simulink model "Udan_SOC"  (R2017b)
settings: Solver=FixedStepAuto  StartTime=0.0  StopTime=1000  FixedStep=0.1  RelTol=1e-3
values from neighbouring files (symbols this model uses):
  DenominatorOfIntegratorFactor = 100.0    [SOC_Stateflow.sldd]
  SOC_CalcSohLKT = 1.0    [SOC_Stateflow.sldd]
  SOC_CalcSOHTempLimit = 70.0    [SOC_Stateflow.sldd]
  SOC_CapPerCycle = 100.0    [SOC_Stateflow.sldd]
  SOC_CapTemp_HLimit = 200.0    [SOC_Stateflow.sldd]
  SOC_CapTemp_LLimit = 0.0    [SOC_Stateflow.sldd]
  Soc_ConfigInfo = 0    [SOC_Stateflow.sldd]
  SOC_DchgEndCalib = 0.0    [SOC_Stateflow.sldd]
  SOC_DiffVoltMin = 10.0    [SOC_Stateflow.sldd]
  SOC_DSOCJumpMax = 500.0    [SOC_Stateflow.sldd]
  SOC_EfficientHighLimit = 250.0    [SOC_Stateflow.sldd]
  SOC_EfficientLowLimit = 40.0    [SOC_Stateflow.sldd]
  SOC_EmptyAus = 0.0    [SOC_Stateflow.sldd]
  SOC_EnableOcv = 1.0    [SOC_Stateflow.sldd]
  SOC_END_CALIB_STATE : value not decoded    [SOC_Stateflow.sldd]
  SOC_HighRealSoc = 95.0    [SOC_Stateflow.sldd]
  SOC_LKTSohCycles = 0.0 1.0 10.0 20.0 30.0 40.0 50.0 60.0 70.0 80.0 90.0 100.0 110.0 120.0 130.0 140.0 150.0 160.0 170.0 180.0 190.0 200.0 210.0 220.0 230.0 240.0 250.0 260.0 270.0 280.0 290.0 300.0 310.0 320.0 330.0 340.0 350.0 360.0 370.0 380.0 390.0 400.0 410.0 420.0 430.0 440.0 450.0 460.0 470.0 480.0 490.0 500.0 510.0 520.0 530.0 540.0 550.0 560.0 570.0 580.0 590.0 600.0 610.0 620.0 630.0 640.0 650.0 660.0 670.0    [SOC_Stateflow.sldd]
  SOC_LKTSohTable = 1000.0 991.0 989.0 992.0 993.0 995.0 994.0 993.0 1000.0 997.0 1002.0 1000.0 992.0 1000.0 989.0 992.0 989.0 994.0 989.0 993.0 994.0 994.0 994.0 993.0 991.0 991.0 992.0 993.0 991.0 985.0 985.0 985.0 979.0 975.0 978.0 984.0 982.0 974.0 975.0 972.0 972.0 975.0 977.0 977.0 974.0 971.0 973.0 971.0 966.0 968.0 965.0 959.0 957.0 956.0 957.0 954.0 955.0 951.0 954.0 951.0 942.0 942.0 940.0 942.0 947.0 949.0    [SOC_Stateflow.sldd]
  SOC_LowRealSoc = 5.0    [SOC_Stateflow.sldd]
  SOC_NominalCap_AmS = 576000000.0    [SOC_Stateflow.sldd]
  SOC_NominalVol = 4000.0    [SOC_Stateflow.sldd]
  SOC_OCVTemp_HLimit = 106.0    [SOC_Stateflow.sldd]
  SOC_OCVTemp_LLimit = 29.0    [SOC_Stateflow.sldd]
  SOC_ShortCalibDSoc = 1.0    [SOC_Stateflow.sldd]
  SOC_SOCResolution = 10000.0    [SOC_Stateflow.sldd]
  SOC_SohCalcCapPercent = 8.0    [SOC_Stateflow.sldd]
  SOC_SohCalcHighLimit = 60.0    [SOC_Stateflow.sldd]
  SOC_SohCalcLowLimit = 10.0    [SOC_Stateflow.sldd]
  SOC_SohCalcMidLimit = 30.0    [SOC_Stateflow.sldd]
  SOC_SOHResolution = 1000.0    [SOC_Stateflow.sldd]
  SOC_State = <binary blob, 1163 chars, not shown>    [SOC_Stateflow.sldd]
  SOC_TempCap_CapBuffer : value not decoded    [SOC_Stateflow.sldd]
  SOC_TempCap_TempBuffer : value not decoded    [SOC_Stateflow.sldd]
  SocOcvCalib_ConfigInfo = 0.0    [SOC_Stateflow.sldd]
  SocOcvCalib_SocBuffer1 : value not decoded    [SOC_Stateflow.sldd]
  SocOcvCalib_TempBuffer : value not decoded    [SOC_Stateflow.sldd]
  SocOcvCalib_VoltageBuffer1 = 3300.0 3303.0 3305.0 3307.0 3310.0 3311.0 3313.0 3314.0 3316.0 3317.0 3319.0 3320.0 3322.0 3323.0 3325.0 3322.0 3323.0 3325.0 3310.0 3313.0 3315.0 3317.0 3320.0 3321.0 3323.0 3324.0 3326.0 3327.0 3329.0 3330.0 3332.0 3333.0 3335.0 3332.0 3333.0 3335.0 3320.0 3323.0 3325.0 3327.0 3330.0 3331.0 3333.0 3334.0 3336.0 3337.0 3339.0 3340.0 3342.0 3343.0 3345.0 3342.0 3343.0 3345.0 3330.0 3333.0 3335.0 3    [SOC_Stateflow.sldd]
  SOHCalibCycle = 10.0    [SOC_Stateflow.sldd]
undefined symbols (not defined in the file or in its folder): DatetimeM_GetReturnType, ParameterM_EeepParaIndexType, Soc_CumuLativeTypeType, SOC_EgthTempChgValue, Soc_EnergyBuffer, SOC_FithTempChgValue, SOC_FstSlowTempChgValue, SOC_FstTempChgValue, SOC_FthTempChgValue, SOC_MaxCap_AmS, SOC_SethTempChgValue, SOC_SixTempChgValue, SOC_SndSlowTempChgValue, SOC_SndTempChgValue, SOC_TrdSlowTempChgValue, SOC_TrdTempChgValue, SocDiagCalib_NoCalibReasonType
libraries: simulink x138, hdlsllib x24, dspindex x4
(part 8 of 10)

== system Udan_SOC/SOC_Calculate/UdanSOCCalcn/WriteSOH/Enabled Subsystem4 ==
  index : Inport
  data : Inport  Port=2
  Enable : EnablePort
  Abs : Abs
  Add : Sum  Inputs=+-  AccumDataTypeStr=int32  OutDataTypeStr=int32
  Constant : Constant  Value=20  OutDataTypeStr=uint8
  Divide : Product  Inputs=*/  OutDataTypeStr=uint32
  Logical Operator : Logic  Operator=OR  AllPortsSameDT=off  OutDataTypeStr=boolean
  Relational Operator : RelationalOperator  OutDataTypeStr=boolean  RndMeth=Simplest
  S-Function1 : S-Function  FunctionName=sfn_NVMRead  SFunctionDeploymentMode=off  EnableBusSupport=off
  EeepWriteFailure : Outport
  wires:
  index/1 -> S-Function1/1
  Logical Operator/1 -> EeepWriteFailure/1
  Abs/1 -> Relational Operator/1
  Relational Operator/1 -> Logical Operator/2
  Constant/1 -> Divide/2
  S-Function1/2 -> Add/1
  Add/1 -> Abs/1
  Divide/1 -> Relational Operator/2
  data/1 -> Divide/1, Add/2
  S-Function1/1 -> Logical Operator/1

== system Udan_SOC/SOC_Calculate/UdanSOCCalcn/WriteSOH/Enabled Subsystem5 ==
  index : Inport
  data : Inport  Port=2
  Enable : EnablePort
  Abs : Abs
  Add : Sum  Inputs=+-  AccumDataTypeStr=int32  OutDataTypeStr=int32
  Constant : Constant  Value=20  OutDataTypeStr=uint8
  Divide : Product  Inputs=*/  OutDataTypeStr=uint32
  Logical Operator : Logic  Operator=OR  AllPortsSameDT=off  OutDataTypeStr=boolean
  Relational Operator : RelationalOperator  OutDataTypeStr=boolean  RndMeth=Simplest
  S-Function1 : S-Function  FunctionName=sfn_NVMRead  SFunctionDeploymentMode=off  EnableBusSupport=off
  EeepWriteFailure : Outport
  wires:
  index/1 -> S-Function1/1
  Logical Operator/1 -> EeepWriteFailure/1
  Abs/1 -> Relational Operator/1
  Relational Operator/1 -> Logical Operator/2
  Constant/1 -> Divide/2
  S-Function1/2 -> Add/1
  Add/1 -> Abs/1
  Divide/1 -> Relational Operator/2
  data/1 -> Divide/1, Add/2
  S-Function1/1 -> Logical Operator/1

== system Udan_SOC/SOC_Calculate/UdanSOCCalcn/WriteSOH/Enabled Subsystem6 ==
  index : Inport
  data : Inport  Port=2
  Enable : EnablePort
  Abs : Abs
  Add : Sum  Inputs=+-  AccumDataTypeStr=int32  OutDataTypeStr=int32
  Constant : Constant  Value=20  OutDataTypeStr=uint8
  Divide : Product  Inputs=*/  OutDataTypeStr=uint32
  Logical Operator : Logic  Operator=OR  AllPortsSameDT=off  OutDataTypeStr=boolean
  Relational Operator : RelationalOperator  OutDataTypeStr=boolean  RndMeth=Simplest
  S-Function1 : S-Function  FunctionName=sfn_NVMRead  SFunctionDeploymentMode=off  EnableBusSupport=off
  EeepWriteFailure : Outport
  wires:
  index/1 -> S-Function1/1
  Logical Operator/1 -> EeepWriteFailure/1
  Abs/1 -> Relational Operator/1
  Relational Operator/1 -> Logical Operator/2
  Constant/1 -> Divide/2
  S-Function1/2 -> Add/1
  Add/1 -> Abs/1
  Divide/1 -> Relational Operator/2
  data/1 -> Divide/1, Add/2
  S-Function1/1 -> Logical Operator/1

== system Udan_SOC/SOC_Calculate/UdanSOCCalcn/WriteSOH/Enabled Subsystem7 ==
  index : Inport
  data : Inport  Port=2
  Enable : EnablePort
  Abs : Abs
  Add : Sum  Inputs=+-  AccumDataTypeStr=int32  OutDataTypeStr=int32
  Constant : Constant  Value=20  OutDataTypeStr=uint8
  Divide : Product  Inputs=*/  OutDataTypeStr=uint32
  Logical Operator : Logic  Operator=OR  AllPortsSameDT=off  OutDataTypeStr=boolean
  Relational Operator : RelationalOperator  OutDataTypeStr=boolean  RndMeth=Simplest
  S-Function1 : S-Function  FunctionName=sfn_NVMRead  SFunctionDeploymentMode=off  EnableBusSupport=off
  EeepWriteFailure : Outport
  wires:
  index/1 -> S-Function1/1
  Logical Operator/1 -> EeepWriteFailure/1
  Abs/1 -> Relational Operator/1
  Relational Operator/1 -> Logical Operator/2
  Constant/1 -> Divide/2
  S-Function1/2 -> Add/1
  Add/1 -> Abs/1
  Divide/1 -> Relational Operator/2
  data/1 -> Divide/1, Add/2
  S-Function1/1 -> Logical Operator/1

== system Udan_SOC/SOC_Calculate/UdanSOCCalcn/CalcChgSOH/Subsystem1/Subsystem ==
  HighIndex : Inport
  LowIndex : Inport  Port=2
  Enable : EnablePort
  Add : Sum
  Bit Rotate : hdlsllib/Logic and Bit Operations/Bit Rotate  mode=Rotate Left  N=16
      settings: SourceProductName=HDL Coder  SourceProductBaseCode=HD
  Data Type Conversion : DataTypeConversion  OutDataTypeStr=uint32
  soc : Outport
  wires:
  LowIndex/1 -> Add/2
  Bit Rotate/1 -> Add/1
  Data Type Conversion/1 -> Bit Rotate/1
  HighIndex/1 -> Data Type Conversion/1
  Add/1 -> soc/1  "soc"

== system Udan_SOC/SOC_Calculate/UdanSOCCalcn/CalcDchgSOH/Subsystem1/Subsystem ==
  HighIndex : Inport
  LowIndex : Inport  Port=2
  Enable : EnablePort
  Add : Sum
  Bit Rotate : hdlsllib/Logic and Bit Operations/Bit Rotate  mode=Rotate Left  N=16
      settings: SourceProductName=HDL Coder  SourceProductBaseCode=HD
  Data Type Conversion : DataTypeConversion  OutDataTypeStr=uint32
  soc : Outport
  wires:
  LowIndex/1 -> Add/2
  Bit Rotate/1 -> Add/1
  Data Type Conversion/1 -> Bit Rotate/1
  HighIndex/1 -> Data Type Conversion/1
  Add/1 -> soc/1  "soc"

== system Udan_SOC/SOC_Calculate/UdanSOCCalcn/CapAdder1/Enabled Subsystem1/Enabled Subsystem1 ==
  CellLowTemp : Inport
  UCell : Inport  Port=2
  CalcSoc : Inport  Port=3
  soh : Inport  Port=4
  Enable : EnablePort
  CalcLeftCap : Subsystem
  Constant11 : Constant  Value=SocOcvCalib_VoltageBuffer1
  Constant12 : Constant  Value=SocOcvCalib_SocBuffer1
  Constant2 : Constant  Value=20  OutDataTypeStr=uint16
  Constant3 : Constant  Value=SocOcvCalib_TempBuffer  OutDataTypeStr=uint8
  Constant6 : Constant  Value=92160  OutDataTypeStr=uint32
  Logical Operator : Logic  Operator=NOT  AllPortsSameDT=off  OutDataTypeStr=boolean
  Lookup Table Dynamic1 : simulink/Lookup Tables/Lookup Table Dynamic  LookUpMeth=Interpolation-Use End Values  OutDataType=fixdt('uint16')  OutScaling=[]  OutputDataTypeScalingMode=Specify via dialog  OutDataTypeStr=uint16  DoSatur=on
      settings: SourceProductName=Simulink
  Lookup Table Dynamic2 : simulink/Lookup Tables/Lookup Table Dynamic  LookUpMeth=Use Input Nearest  OutDataType=fixdt('uint8')  OutScaling=[]  OutputDataTypeScalingMode=Specify via dialog  OutDataTypeStr=uint8  DoSatur=on
      settings: SourceProductName=Simulink
  MATLAB Function : MATLAB Function  TreatAsAtomicUnit=on
  Relational Operator2 : RelationalOperator  OutDataTypeStr=boolean  RndMeth=Simplest
  Switch : Switch  Criteria=u2 > Threshold
  Variable Selector : dspindex/Variable Selector  NumInputs=1  rowsOrCols=Rows  IdxMode=Variable  Elements=[1 3]  ZerOneIdxMode=One-based  errmode=Clip Index  FillMode=on  FillValues=0
  LKTSOC : Outport
  LeftCap2 : Outport  Port=2
  wires:
  CellLowTemp/1 -> Lookup Table Dynamic2/1, CalcLeftCap/2(CellLowTemp)
  UCell/1 -> Lookup Table Dynamic1/1
  Lookup Table Dynamic2/1 -> Variable Selector/2
  MATLAB Function/1(y) -> Lookup Table Dynamic2/3
  Constant3/1 -> MATLAB Function/1(u), Lookup Table Dynamic2/2
  Constant12/1 -> Lookup Table Dynamic1/3
  Variable Selector/1 -> Lookup Table Dynamic1/2
  Lookup Table Dynamic1/1 -> LKTSOC/1, CalcLeftCap/1(soc), Relational Operator2/1  "soc"
  Relational Operator2/1 -> Logical Operator/1, CalcLeftCap/Enable
  Switch/1 -> LeftCap2/1
  Constant2/1 -> Relational Operator2/2
  Constant6/1 -> Switch/1  "soc"
  Logical Operator/1 -> Switch/2
  CalcLeftCap/1(Soc) -> Switch/3
  CalcSoc/1 -> CalcLeftCap/3(CalcSoc)
  soh/1 -> CalcLeftCap/4(soh)
  Constant11/1 -> Variable Selector/1

== system Udan_SOC/SOC_Calculate/UdanSOCCalcn/CapAdder1/Enabled Subsystem1/Function-Call Subsystem ==
  function : TriggerPort  TriggerType=function-call  VariantControl=Variant
  sfn_SetLowPower : S-Function  FunctionName=sfn_SetLowPower  SFunctionDeploymentMode=off  EnableBusSupport=off  mask(Legacy Function){SFunctionSpec=void UserSetLowPowerFlg(void), ShowSpec=on}
      mask prompts: ShowSpec "Display function specification"
      mask help:
      | This block allows you to call the legacy functions specified by the following Legacy Code Tool definition:
      | def.SFunctionName = 'sfn_SetLowPower';
      | def.OutputFcnSpec = 'void UserSetLowPowerFlg(void)';
      | def.HeaderFiles = {'PowerM.h'};
      mask Help: <p>This block was generated automatically by the Legacy Code Tool. For detailed help on this tool, call<a href="matlab:legacy_code('help')"> legacy_code('help')</a>.</p>
      mask Callback ShowSpec:
      | if strcmp(get_param(gcbh, 'ShowSpec'), 'on')
      |   set_param(gcbh, 'MaskDisplay', sprintf('fprintf(''%s'');', get_param(gcbh, 'SFunctionSpec')));
      | else
      |   set_param(gcbh, 'MaskDisplay', sprintf('fprintf(''%s'');', get_param(gcbh, 'FunctionName')));
      | end
      mask Display: fprintf('void UserSetLowPowerFlg(void)');

== system Udan_SOC/SOC_Calculate/UdanSOCCalcn/CapAdder1/LKT/LKT_Temp20 ==
  Cur : Inport
  UCell : Inport  Port=2
  Enable : EnablePort
  Constant : Constant  Value=1000  OutDataTypeStr=uint16
  Constant1 : Constant  Value=1000  OutDataTypeStr=uint16
  Constant2 : Constant  Value=500  OutDataTypeStr=uint16
  Constant3 : Constant  Value=0  OutDataTypeStr=uint8
  Current_1C : Subsystem  TreatAsAtomicUnit=on
  Current_1C1 : Subsystem  TreatAsAtomicUnit=on
  Logical Operator : Logic  AllPortsSameDT=off  OutDataTypeStr=boolean
  Logical Operator1 : Logic  Operator=NOT  AllPortsSameDT=off  OutDataTypeStr=boolean
  Logical Operator2 : Logic  Operator=NOT  AllPortsSameDT=off  OutDataTypeStr=boolean
  Relational Operator : RelationalOperator  OutDataTypeStr=boolean  RndMeth=Simplest
  Relational Operator1 : RelationalOperator  Operator=<  OutDataTypeStr=boolean  RndMeth=Simplest
  Relational Operator2 : RelationalOperator  OutDataTypeStr=boolean  RndMeth=Simplest
  Switch : Switch  Criteria=u2 > Threshold
  Switch1 : Switch  Criteria=u2 > Threshold
  SOC : Outport
  wires:
  Constant/1 -> Relational Operator/2
  Relational Operator/1 -> Logical Operator2/1, Current_1C/Enable
  UCell/1 -> Current_1C1/1(UCell), Current_1C/1(UCell)
  Constant1/1 -> Relational Operator1/2
  Constant2/1 -> Relational Operator2/2
  Relational Operator1/1 -> Logical Operator/1
  Relational Operator2/1 -> Logical Operator/2
  Logical Operator/1 -> Logical Operator1/1, Current_1C1/Enable
  Cur/1 -> Relational Operator/1, Relational Operator1/1, Relational Operator2/1
  Logical Operator1/1 -> Switch/2
  Current_1C1/1(SOC) -> Switch/3
  Logical Operator2/1 -> Switch1/2
  Current_1C/1(SOC) -> Switch1/3
  Switch1/1 -> Switch/1
  Constant3/1 -> Switch1/1
  Switch/1 -> SOC/1

== system Udan_SOC/SOC_Calculate/UdanSOCCalcn/CapAdder1/LKT/LKT_Temp40 ==
  Cur : Inport
  UCell : Inport  Port=2
  Enable : EnablePort
  Constant1 : Constant  Value=500  OutDataTypeStr=uint16
  Constant2 : Constant  Value=200  OutDataTypeStr=uint16
  Constant3 : Constant  Value=500  OutDataTypeStr=uint16
  Constant4 : Constant  Value=0  OutDataTypeStr=uint8
  Constant6 : Constant  Value=4118  OutDataTypeStr=uint16
  Current_1C : Subsystem  TreatAsAtomicUnit=on
  Current_1C1 : Subsystem  TreatAsAtomicUnit=on
  Logical Operator : Logic  Inputs=3  AllPortsSameDT=off  OutDataTypeStr=boolean
  Logical Operator1 : Logic  Operator=NOT  AllPortsSameDT=off  OutDataTypeStr=boolean
  Logical Operator2 : Logic  Operator=NOT  AllPortsSameDT=off  OutDataTypeStr=boolean
  Relational Operator1 : RelationalOperator  Operator=<  OutDataTypeStr=boolean  RndMeth=Simplest
  Relational Operator2 : RelationalOperator  OutDataTypeStr=boolean  RndMeth=Simplest
  Relational Operator3 : RelationalOperator  OutDataTypeStr=boolean  RndMeth=Simplest
  Relational Operator4 : RelationalOperator  OutDataTypeStr=boolean  RndMeth=Simplest
  Switch : Switch  Criteria=u2 > Threshold
  Switch1 : Switch  Criteria=u2 > Threshold
  SOC : Outport
  wires:
  Cur/1 -> Relational Operator1/1, Relational Operator2/1, Relational Operator3/1
  Constant1/1 -> Relational Operator1/2
  Relational Operator2/1 -> Logical Operator/2
  Relational Operator1/1 -> Logical Operator/1
  Constant2/1 -> Relational Operator2/2
  Constant3/1 -> Relational Operator3/2
  Relational Operator3/1 -> Logical Operator2/1, Current_1C/Enable
  UCell/1 -> Current_1C1/1(UCell), Relational Operator4/1, Current_1C/1(UCell)
  Logical Operator1/1 -> Switch/2
  Switch1/1 -> Switch/1
  Switch/1 -> SOC/1
  Constant4/1 -> Switch1/1
  Current_1C/1(SOC) -> Switch1/3
  Current_1C1/1(SOC) -> Switch/3
  Logical Operator2/1 -> Switch1/2
  Logical Operator/1 -> Logical Operator1/1, Current_1C1/Enable
  Constant6/1 -> Relational Operator4/2
  Relational Operator4/1 -> Logical Operator/3

== system Udan_SOC/SOC_Calculate/UdanSOCCalcn/CapAdder1/LKT/LKT_Temp45 ==
  Cur : Inport
  UCell : Inport  Port=2
  Enable : EnablePort
  Constant1 : Constant  Value=175  OutDataTypeStr=uint16
  Constant2 : Constant  Value=100  OutDataTypeStr=uint16
  Constant3 : Constant  Value=250  OutDataTypeStr=uint16
  Constant4 : Constant  Value=0  OutDataTypeStr=uint8
  Current_1C : Subsystem  TreatAsAtomicUnit=on
  Current_1C1 : Subsystem  TreatAsAtomicUnit=on
  Logical Operator : Logic  AllPortsSameDT=off  OutDataTypeStr=boolean
  Logical Operator1 : Logic  Operator=NOT  AllPortsSameDT=off  OutDataTypeStr=boolean
  Logical Operator2 : Logic  Operator=NOT  AllPortsSameDT=off  OutDataTypeStr=boolean
  Relational Operator1 : RelationalOperator  Operator=<  OutDataTypeStr=boolean  RndMeth=Simplest
  Relational Operator2 : RelationalOperator  OutDataTypeStr=boolean  RndMeth=Simplest
  Relational Operator3 : RelationalOperator  Operator=>  OutDataTypeStr=boolean  RndMeth=Simplest
  Switch : Switch  Criteria=u2 > Threshold
  Switch1 : Switch  Criteria=u2 > Threshold
  SOC : Outport
  wires:
  Relational Operator3/1 -> Logical Operator2/1, Current_1C/Enable
  UCell/1 -> Current_1C1/1(UCell), Current_1C/1(UCell)
  Cur/1 -> Relational Operator2/1, Relational Operator1/1, Relational Operator3/1
  Constant3/1 -> Relational Operator3/2
  Current_1C/1(SOC) -> Switch1/3
  Current_1C1/1(SOC) -> Switch/3
  Constant1/1 -> Relational Operator1/2
  Relational Operator2/1 -> Logical Operator/2
  Switch/1 -> SOC/1
  Logical Operator/1 -> Logical Operator1/1, Current_1C1/Enable
  Constant4/1 -> Switch1/1
  Logical Operator1/1 -> Switch/2
  Switch1/1 -> Switch/1
  Relational Operator1/1 -> Logical Operator/1
  Logical Operator2/1 -> Switch1/2
  Constant2/1 -> Relational Operator2/2

== system Udan_SOC/SOC_Calculate/UdanSOCCalcn/Function-Call Subsystem4/Subsystem1/Subsystem ==
  HighIndex : Inport
  LowIndex : Inport  Port=2
  Enable : EnablePort
  Add : Sum
  Bit Rotate : hdlsllib/Logic and Bit Operations/Bit Rotate  mode=Rotate Left  N=16
      settings: SourceProductName=HDL Coder  SourceProductBaseCode=HD
  Data Type Conversion : DataTypeConversion  OutDataTypeStr=uint32
  soc : Outport
  wires:
  LowIndex/1 -> Add/2
  Bit Rotate/1 -> Add/1
  Data Type Conversion/1 -> Bit Rotate/1
  HighIndex/1 -> Data Type Conversion/1
  Add/1 -> soc/1  "soc"

== system Udan_SOC/SOC_Calculate/UdanSOCCalcn/Function-Call Subsystem4/Subsystem1/Subsystem1 ==
  HighIndex : Inport
  LowIndex : Inport  Port=2
  DefaultValue : Inport  Port=3
  Enable : EnablePort
  Constant1 : Constant  Value=0  OutDataTypeStr=uint8
  Constant2 : Constant  Value=0  OutDataTypeStr=uint8
  Logical Operator : Logic  AllPortsSameDT=off  OutDataTypeStr=boolean
  Logical Operator1 : Logic  Operator=NOT  AllPortsSameDT=off  OutDataTypeStr=boolean
  Relational Operator : RelationalOperator  Operator===  OutDataTypeStr=boolean  RndMeth=Simplest
  Relational Operator1 : RelationalOperator  Operator===  OutDataTypeStr=boolean  RndMeth=Simplest
  S-Function : S-Function  FunctionName=sfn_NVMRead  SFunctionDeploymentMode=off  EnableBusSupport=off
  S-Function1 : S-Function  FunctionName=sfn_NVMRead  SFunctionDeploymentMode=off  EnableBusSupport=off
  Subsystem : Subsystem
  Switch : Switch  Criteria=u2 > Threshold
  EeepRead32 : Outport
  wires:
  DefaultValue/1 -> Switch/1
  [ReadLowOk] -> Logical Operator/1
  S-Function/2 -> Subsystem/1(HighIndex)
  S-Function/1 -> Relational Operator/1
  S-Function1/2 -> Subsystem/2(LowIndex)
  HighIndex/1 -> S-Function/1
  Constant1/1 -> Relational Operator/2
  Constant2/1 -> Relational Operator1/2
  LowIndex/1 -> S-Function1/1
  Relational Operator/1 -> Logical Operator/2
  Logical Operator/1 -> Logical Operator1/1, Subsystem/Enable
  Relational Operator1/1 -> [ReadLowOk]
  S-Function1/1 -> Relational Operator1/1
  Subsystem/1(soc) -> Switch/3
  Logical Operator1/1 -> Switch/2
  Switch/1 -> EeepRead32/1

== system Udan_SOC/SOC_Calculate/UdanSOCCalcn/Function-Call Subsystem4/Subsystem2/Subsystem ==
  data : Inport
  HighIndex : Inport  Port=2
  LowIndex : Inport  Port=3
  Bit Rotate : hdlsllib/Logic and Bit Operations/Bit Rotate  mode=Rotate Right  N=16
      settings: SourceProductName=HDL Coder  SourceProductBaseCode=HD
  Data Type Conversion : DataTypeConversion  OutDataTypeStr=uint16
  Data Type Conversion1 : DataTypeConversion  OutDataTypeStr=uint16
  S-Function : S-Function  FunctionName=sfn_NVMWrite  SFunctionDeploymentMode=off  EnableBusSupport=off
  S-Function1 : S-Function  FunctionName=sfn_NVMWrite  SFunctionDeploymentMode=off  EnableBusSupport=off
  Terminator : Terminator
  Terminator1 : Terminator
  wires:
  data/1 -> Data Type Conversion1/1, Bit Rotate/1
  Data Type Conversion/1 -> S-Function/2
  S-Function1/1 -> Terminator1/1
  Bit Rotate/1 -> Data Type Conversion/1
  Data Type Conversion1/1 -> S-Function1/2
  S-Function/1 -> Terminator/1
  HighIndex/1 -> S-Function/1
  LowIndex/1 -> S-Function1/1

== system Udan_SOC/SOC_Calculate/UdanSOCCalcn/LKTSOC/Subsystem1/Subsystem ==
  HighIndex : Inport
  LowIndex : Inport  Port=2
  Enable : EnablePort
  Add : Sum
  Bit Rotate : hdlsllib/Logic and Bit Operations/Bit Rotate  mode=Rotate Left  N=16
      settings: SourceProductName=HDL Coder  SourceProductBaseCode=HD
  Data Type Conversion : DataTypeConversion  OutDataTypeStr=uint32
  soc : Outport
  wires:
  LowIndex/1 -> Add/2
  Bit Rotate/1 -> Add/1
  Data Type Conversion/1 -> Bit Rotate/1
  HighIndex/1 -> Data Type Conversion/1
  Add/1 -> soc/1  "soc"

== system Udan_SOC/SOC_Calculate/UdanSOCCalcn/StoreCulumutiveAh/StoreChgAh/Subsystem ==
  data : Inport
  HighIndex : Inport  Port=2
  LowIndex : Inport  Port=3
  Bit Rotate : hdlsllib/Logic and Bit Operations/Bit Rotate  mode=Rotate Right  N=16
      settings: SourceProductName=HDL Coder  SourceProductBaseCode=HD
  Data Type Conversion : DataTypeConversion  OutDataTypeStr=uint16
  Data Type Conversion1 : DataTypeConversion  OutDataTypeStr=uint16
  S-Function : S-Function  FunctionName=sfn_NVMWrite  SFunctionDeploymentMode=off  EnableBusSupport=off
  S-Function1 : S-Function  FunctionName=sfn_NVMWrite  SFunctionDeploymentMode=off  EnableBusSupport=off
  Terminator : Terminator
  Terminator1 : Terminator
  wires:
  data/1 -> Data Type Conversion1/1, Bit Rotate/1
  Data Type Conversion/1 -> S-Function/2
  S-Function1/1 -> Terminator1/1
  Bit Rotate/1 -> Data Type Conversion/1
  Data Type Conversion1/1 -> S-Function1/2
  S-Function/1 -> Terminator/1
  HighIndex/1 -> S-Function/1
  LowIndex/1 -> S-Function1/1

== system Udan_SOC/SOC_Calculate/UdanSOCCalcn/StoreCulumutiveAh/StoreChgAh/Subsystem1 ==
  HighIndex : Inport
  LowIndex : Inport  Port=2
  DefaultValue : Inport  Port=3
  Constant1 : Constant  Value=0  OutDataTypeStr=uint8
  Constant2 : Constant  Value=0  OutDataTypeStr=uint8
  Logical Operator : Logic  AllPortsSameDT=off  OutDataTypeStr=boolean
  Logical Operator1 : Logic  Operator=NOT  AllPortsSameDT=off  OutDataTypeStr=boolean
  Relational Operator : RelationalOperator  Operator===  OutDataTypeStr=boolean  RndMeth=Simplest
  Relational Operator1 : RelationalOperator  Operator===  OutDataTypeStr=boolean  RndMeth=Simplest
  S-Function : S-Function  FunctionName=sfn_NVMRead  SFunctionDeploymentMode=off  EnableBusSupport=off
  S-Function1 : S-Function  FunctionName=sfn_NVMRead  SFunctionDeploymentMode=off  EnableBusSupport=off
  Subsystem : Subsystem
  Switch : Switch  Criteria=u2 > Threshold
  EeepRead32 : Outport
  wires:
  DefaultValue/1 -> Switch/1
  [ReadLowOk] -> Logical Operator/1
  S-Function/2 -> Subsystem/1(HighIndex)
  S-Function/1 -> Relational Operator/1
  S-Function1/2 -> Subsystem/2(LowIndex)
  HighIndex/1 -> S-Function/1
  Constant1/1 -> Relational Operator/2
  Constant2/1 -> Relational Operator1/2
  LowIndex/1 -> S-Function1/1
  Relational Operator/1 -> Logical Operator/2
  Logical Operator/1 -> Logical Operator1/1, Subsystem/Enable
  Relational Operator1/1 -> [ReadLowOk]
  S-Function1/1 -> Relational Operator1/1
  Subsystem/1(soc) -> Switch/3
  Logical Operator1/1 -> Switch/2
  Switch/1 -> EeepRead32/1

== system Udan_SOC/SOC_Calculate/UdanSOCCalcn/StoreCulumutiveAh/StoreDchgAh1/Subsystem ==
  data : Inport
  HighIndex : Inport  Port=2
  LowIndex : Inport  Port=3
  Bit Rotate : hdlsllib/Logic and Bit Operations/Bit Rotate  mode=Rotate Right  N=16
      settings: SourceProductName=HDL Coder  SourceProductBaseCode=HD
  Data Type Conversion : DataTypeConversion  OutDataTypeStr=uint16
  Data Type Conversion1 : DataTypeConversion  OutDataTypeStr=uint16
  S-Function : S-Function  FunctionName=sfn_NVMWrite  SFunctionDeploymentMode=off  EnableBusSupport=off
  S-Function1 : S-Function  FunctionName=sfn_NVMWrite  SFunctionDeploymentMode=off  EnableBusSupport=off
  Terminator : Terminator
  Terminator1 : Terminator
  wires:
  data/1 -> Data Type Conversion1/1, Bit Rotate/1
  Data Type Conversion/1 -> S-Function/2
  S-Function1/1 -> Terminator1/1
  Bit Rotate/1 -> Data Type Conversion/1
  Data Type Conversion1/1 -> S-Function1/2
  S-Function/1 -> Terminator/1
  HighIndex/1 -> S-Function/1
  LowIndex/1 -> S-Function1/1

== system Udan_SOC/SOC_Calculate/UdanSOCCalcn/StoreCulumutiveAh/StoreDchgAh1/Subsystem1 ==
  HighIndex : Inport
  LowIndex : Inport  Port=2
  DefaultValue : Inport  Port=3
  Constant1 : Constant  Value=0  OutDataTypeStr=uint8
  Constant2 : Constant  Value=0  OutDataTypeStr=uint8
  Logical Operator : Logic  AllPortsSameDT=off  OutDataTypeStr=boolean
  Logical Operator1 : Logic  Operator=NOT  AllPortsSameDT=off  OutDataTypeStr=boolean
  Relational Operator : RelationalOperator  Operator===  OutDataTypeStr=boolean  RndMeth=Simplest
  Relational Operator1 : RelationalOperator  Operator===  OutDataTypeStr=boolean  RndMeth=Simplest
  S-Function : S-Function  FunctionName=sfn_NVMRead  SFunctionDeploymentMode=off  EnableBusSupport=off
  S-Function1 : S-Function  FunctionName=sfn_NVMRead  SFunctionDeploymentMode=off  EnableBusSupport=off
  Subsystem : Subsystem
  Switch : Switch  Criteria=u2 > Threshold
  EeepRead32 : Outport
  wires:
  DefaultValue/1 -> Switch/1
  [ReadLowOk] -> Logical Operator/1
  S-Function/2 -> Subsystem/1(HighIndex)
  S-Function/1 -> Relational Operator/1
  S-Function1/2 -> Subsystem/2(LowIndex)
  HighIndex/1 -> S-Function/1
  Constant1/1 -> Relational Operator/2
  Constant2/1 -> Relational Operator1/2
  LowIndex/1 -> S-Function1/1
  Relational Operator/1 -> Logical Operator/2
  Logical Operator/1 -> Logical Operator1/1, Subsystem/Enable
  Relational Operator1/1 -> [ReadLowOk]
  S-Function1/1 -> Relational Operator1/1
  Subsystem/1(soc) -> Switch/3
  Logical Operator1/1 -> Switch/2
  Switch/1 -> EeepRead32/1

== system Udan_SOC/SOC_Calculate/UdanSOCCalcn/StoreLeftCap/WriteLeftCap/Subsystem ==
  data : Inport
  HighIndex : Inport  Port=2
  LowIndex : Inport  Port=3
  Bit Rotate : hdlsllib/Logic and Bit Operations/Bit Rotate  mode=Rotate Right  N=16
      settings: SourceProductName=HDL Coder  SourceProductBaseCode=HD
  Data Type Conversion : DataTypeConversion  OutDataTypeStr=uint16
  Data Type Conversion1 : DataTypeConversion  OutDataTypeStr=uint16
  Logical Operator : Logic  Operator=OR  AllPortsSameDT=off  OutDataTypeStr=boolean
  S-Function : S-Function  FunctionName=sfn_NVMWrite  SFunctionDeploymentMode=off  EnableBusSupport=off
  S-Function1 : S-Function  FunctionName=sfn_NVMWrite  SFunctionDeploymentMode=off  EnableBusSupport=off
  Terminator : Terminator
  wires:
  data/1 -> Data Type Conversion1/1, Bit Rotate/1
  Data Type Conversion/1 -> S-Function/2
  S-Function1/1 -> Logical Operator/2
  Bit Rotate/1 -> Data Type Conversion/1
  Data Type Conversion1/1 -> S-Function1/2
  S-Function/1 -> Logical Operator/1
  HighIndex/1 -> S-Function/1
  LowIndex/1 -> S-Function1/1
  Logical Operator/1 -> Terminator/1

== system Udan_SOC/SOC_Calculate/UdanSOCCalcn/StoreSOC/Subsystem/Enabled Subsystem1 ==
  Enable : EnablePort
  Add : Sum  Inputs=+++  OutDataTypeStr=uint32
  Bit Rotate1 : hdlsllib/Logic and Bit Operations/Bit Rotate  mode=Rotate Right  N=16
      settings: SourceProductName=HDL Coder  SourceProductBaseCode=HD
  Bit Rotate2 : hdlsllib/Logic and Bit Operations/Bit Rotate  mode=Rotate Left  N=16
      settings: SourceProductName=HDL Coder  SourceProductBaseCode=HD
  Constant16 : Constant  Value=SOC_NominalCap_AmS
  Constant5 : Constant  Value=350  OutDataTypeStr=uint16
  Data Type Conversion : DataTypeConversion  OutDataTypeStr=uint16
  Data Type Conversion1 : DataTypeConversion  OutDataTypeStr=uint16
  Data Type Conversion2 : DataTypeConversion  OutDataTypeStr=uint32
  DchgPower1 : simulink/Sources/Enumerated Constant  OutDataTypeStr=Enum: ParameterM_EeepParaIndexType  Value=ParameterM_EeepParaIndexType.PARAMETERM_EEEP_LEFTCAP_WOCALIB_H_INDEX  SampleTime=inf
      settings: SourceProductName=Simulink
  DchgPower2 : simulink/Sources/Enumerated Constant  OutDataTypeStr=Enum: ParameterM_EeepParaIndexType  Value=ParameterM_EeepParaIndexType.PARAMETERM_EEEP_LEFTCAP_WOCALIB_L_INDEX  SampleTime=inf
      settings: SourceProductName=Simulink
  DchgPower3 : simulink/Sources/Enumerated Constant  OutDataTypeStr=Enum: ParameterM_EeepParaIndexType  Value=ParameterM_EeepParaIndexType.PARAMETERM_EEEP_LEFTCAP_WOCALIB_H_INDEX  SampleTime=inf
      settings: SourceProductName=Simulink
  DchgPower4 : simulink/Sources/Enumerated Constant  OutDataTypeStr=Enum: ParameterM_EeepParaIndexType  Value=ParameterM_EeepParaIndexType.PARAMETERM_EEEP_LEFTCAP_WOCALIB_L_INDEX  SampleTime=inf
      settings: SourceProductName=Simulink
  Divide8 : Product  Inputs=*/  OutDataTypeStr=uint32
  S-Function : S-Function  FunctionName=sfn_NVMWrite  SFunctionDeploymentMode=off  EnableBusSupport=off
  S-Function1 : S-Function  FunctionName=sfn_NVMRead  SFunctionDeploymentMode=off  EnableBusSupport=off
  S-Function2 : S-Function  FunctionName=sfn_NVMWrite  SFunctionDeploymentMode=off  EnableBusSupport=off
  S-Function3 : S-Function  FunctionName=sfn_NVMRead  SFunctionDeploymentMode=off  EnableBusSupport=off
  Terminator{1..4} (4 alike) : Terminator
  wires:
  DchgPower4/1 -> S-Function2/1
  Data Type Conversion/1 -> S-Function/2
  Add/1 -> Bit Rotate1/1, Data Type Conversion1/1
  S-Function2/1 -> Terminator3/1
  DchgPower3/1 -> S-Function/1
  Data Type Conversion1/1 -> S-Function2/2
  S-Function/1 -> Terminator2/1
  Bit Rotate1/1 -> Data Type Conversion/1
  Divide8/1 -> Add/1
  DchgPower1/1 -> S-Function1/1
  S-Function1/2 -> Data Type Conversion2/1
  S-Function1/1 -> Terminator1/1
  DchgPower2/1 -> S-Function3/1
  S-Function3/1 -> Terminator4/1
  S-Function3/2 -> Add/3
  Data Type Conversion2/1 -> Bit Rotate2/1
  Bit Rotate2/1 -> Add/2
  Constant5/1 -> Divide8/2
  Constant16/1 -> Divide8/1

== system Udan_SOC/SOC_Calculate/UdanSOCCalcn/StoreSOC/Subsystem1/Enabled Subsystem1 ==
  Enable : EnablePort
  Add : Sum  Inputs=++-  OutDataTypeStr=int32
  Bit Rotate1 : hdlsllib/Logic and Bit Operations/Bit Rotate  mode=Rotate Right  N=16
      settings: SourceProductName=HDL Coder  SourceProductBaseCode=HD
  Bit Rotate2 : hdlsllib/Logic and Bit Operations/Bit Rotate  mode=Rotate Left  N=16
      settings: SourceProductName=HDL Coder  SourceProductBaseCode=HD
  Constant1 : Constant  Value=0  OutDataTypeStr=uint8
  Constant16 : Constant  Value=SOC_NominalCap_AmS
  Constant31 : Constant  Value=SOC_NominalCap_AmS
  Constant42 : Constant  Value=SOC_SOHResolution  OutDataTypeStr=uint16
  Constant43 : Constant  Value=SOC_TempCap_CapBuffer
  Constant5 : Constant  Value=350  OutDataTypeStr=uint16
  Data Type Conversion : DataTypeConversion  OutDataTypeStr=uint16
  Data Type Conversion1 : DataTypeConversion  OutDataTypeStr=uint16
  Data Type Conversion2 : DataTypeConversion  OutDataTypeStr=uint32
  DchgPower1 : simulink/Sources/Enumerated Constant  OutDataTypeStr=Enum: ParameterM_EeepParaIndexType  Value=ParameterM_EeepParaIndexType.PARAMETERM_EEEP_LEFTCAP_WOCALIB_H_INDEX  SampleTime=inf
      settings: SourceProductName=Simulink
  DchgPower2 : simulink/Sources/Enumerated Constant  OutDataTypeStr=Enum: ParameterM_EeepParaIndexType  Value=ParameterM_EeepParaIndexType.PARAMETERM_EEEP_LEFTCAP_WOCALIB_L_INDEX  SampleTime=inf
      settings: SourceProductName=Simulink
  DchgPower3 : simulink/Sources/Enumerated Constant  OutDataTypeStr=Enum: ParameterM_EeepParaIndexType  Value=ParameterM_EeepParaIndexType.PARAMETERM_EEEP_LEFTCAP_WOCALIB_H_INDEX  SampleTime=inf
      settings: SourceProductName=Simulink
  DchgPower4 : simulink/Sources/Enumerated Constant  OutDataTypeStr=Enum: ParameterM_EeepParaIndexType  Value=ParameterM_EeepParaIndexType.PARAMETERM_EEEP_LEFTCAP_WOCALIB_L_INDEX  SampleTime=inf
      settings: SourceProductName=Simulink
  Divide16 : Product  Inputs=*/*  OutDataTypeStr=uint32
  Divide8 : Product  Inputs=*/  OutDataTypeStr=uint32
  MinMax : MinMax  Function=max
  S-Function : S-Function  FunctionName=sfn_NVMWrite  SFunctionDeploymentMode=off  EnableBusSupport=off
  S-Function1 : S-Function  FunctionName=sfn_NVMRead  SFunctionDeploymentMode=off  EnableBusSupport=off
  S-Function2 : S-Function  FunctionName=sfn_NVMWrite  SFunctionDeploymentMode=off  EnableBusSupport=off
  S-Function3 : S-Function  FunctionName=sfn_NVMRead  SFunctionDeploymentMode=off  EnableBusSupport=off
  Saturation Dynamic : simulink/Discontinuities/Saturation Dynamic  OutMin=[]  OutMax=[]  OutDataTypeStr=uint32  OutputDataTypeScalingMode=uint32  OutDataType=fixdt(1, 16)  OutScaling=2^-10  DoSatur=off
  Terminator{1..4} (4 alike) : Terminator
  wires:
  DchgPower4/1 -> S-Function2/1
  Data Type Conversion/1 -> S-Function/2
  Saturation Dynamic/1 -> Bit Rotate1/1, Data Type Conversion1/1
  S-Function2/1 -> Terminator3/1
  DchgPower3/1 -> S-Function/1
  Data Type Conversion1/1 -> S-Function2/2
  S-Function/1 -> Terminator2/1
  Bit Rotate1/1 -> Data Type Conversion/1
  Divide8/1 -> Add/3
  DchgPower1/1 -> S-Function1/1
  S-Function1/2 -> Data Type Conversion2/1
  S-Function1/1 -> Terminator1/1
  DchgPower2/1 -> S-Function3/1
  S-Function3/1 -> Terminator4/1
  S-Function3/2 -> Add/2
  Data Type Conversion2/1 -> Bit Rotate2/1
  Bit Rotate2/1 -> Add/1
  Constant1/1 -> Saturation Dynamic/3
  Divide16/1 -> Saturation Dynamic/1
  Add/1 -> Saturation Dynamic/2
  Constant5/1 -> Divide8/2
  Constant16/1 -> Divide8/1
  Constant31/1 -> Divide16/1
  Constant43/1 -> MinMax/1
  Constant42/1 -> Divide16/2
  MinMax/1 -> Divide16/3

== system Udan_SOC/SOC_Calculate/UdanSOCCalcn/CapAdder1/Enabled Subsystem1/Enabled Subsystem1/CalcLeftCap ==
  soc : Inport
  CellLowTemp : Inport  Port=2
  CalcSoc : Inport  Port=3
  soh : Inport  Port=4
  Enable : EnablePort
  Add : Sum  OutDataTypeStr=uint32
  Add2 : Sum  Inputs=+-  OutDataTypeStr=int32
  Chart : Stateflow chart  TreatAsAtomicUnit=on
  Constant : Constant  Value=0  OutDataTypeStr=uint8
  Constant1 : Constant  Value=SOC_SOHResolution  OutDataTypeStr=uint16
  Constant10 : Constant  Value=0  OutDataTypeStr=uint8
  Constant2 : Constant  Value=0  OutDataTypeStr=uint16
  Constant22 : Constant  Value=SOC_SOCResolution  OutDataTypeStr=uint16
  Constant25 : Constant  Value=SOC_NominalCap_AmS
  Constant3 : Constant  Value=SOC_SOCResolution  OutDataTypeStr=uint16
  Constant31 : Constant  Value=SOC_NominalCap_AmS
  Constant4 : Constant  Value=SOC_NominalCap_AmS
  Constant42 : Constant  Value=SOC_SOHResolution  OutDataTypeStr=uint16
  Constant43 : Constant  Value=SOC_TempCap_CapBuffer
  Constant5 : Constant  Value=10000  OutDataTypeStr=uint16
  Constant6 : Constant  Value=691200000  OutDataTypeStr=uint32
  Constant8 : Constant  Value=SOC_SOHResolution  OutDataTypeStr=uint16
  Divide : Product  Inputs=*/*  OutDataTypeStr=uint32
  Divide1 : Product  Inputs=*/*  OutDataTypeStr=uint32
  Divide16 : Product  Inputs=*/*  OutDataTypeStr=uint32
  Divide2 : Product  Inputs=**  OutDataTypeStr=uint32
  Divide3 : Product  Inputs=*/  OutDataTypeStr=int32
  Divide4 : Product  Inputs=*/  OutDataTypeStr=uint32
  Divide5 : Product  Inputs=*/  OutDataTypeStr=uint32
  MinMax : MinMax  Function=max
  MinMax1 : MinMax  Function=max  Inputs=2
  Saturation Dynamic : simulink/Discontinuities/Saturation Dynamic  OutMin=[]  OutMax=[]  OutDataTypeStr=Inherit: Same as second input  OutDataType=fixdt(1, 16)  OutScaling=2^-10  DoSatur=off
  Saturation Dynamic1 : simulink/Discontinuities/Saturation Dynamic  OutMin=[]  OutMax=[]  OutDataTypeStr=uint32  OutputDataTypeScalingMode=uint32  OutDataType=fixdt(1, 16)  OutScaling=2^-10  DoSatur=on
  Saturation Dynamic2 : simulink/Discontinuities/Saturation Dynamic  OutMin=[]  OutMax=[]  OutDataTypeStr=Inherit: Same as second input  OutDataType=fixdt(1, 16)  OutScaling=2^-10  DoSatur=off
  Subtract : Sum  Inputs=+-  AccumDataTypeStr=int32  OutDataTypeStr=int32
  TempCapTable1 : Lookup_n-D  NumberOfTableDimensions=1  BreakpointsForDimension1=SOC_TempCap_TempBuffer  Table=SOC_TempCap_CapBuffer  ExtrapMethod=Clip  InternalRulePriority=Speed  OutDataTypeStr=uint16  RndMeth=Simplest  InputSameDT=on
  Soc : Outport  InitialOutput=0
  wires:
  Divide1/1 -> Saturation Dynamic/2
  soc/1 -> [soc]
  Constant22/1 -> Divide/2
  Add/1 -> Divide1/1
  Saturation Dynamic/1 -> Soc/1  "soc"
  Constant2/1 -> Saturation Dynamic/3
  Divide/1 -> Add/2
  CellLowTemp/1 -> TempCapTable1/1
  Constant6/1 -> Saturation Dynamic/1
  Saturation Dynamic2/1 -> Divide/1, [TCap], Add2/2
  TempCapTable1/1 -> Divide2/1
  Constant8/1 -> Divide1/2
  CalcSoc/1 -> Subtract/1
  [CannotUsedCap] -> Subtract/2
  Subtract/1 -> Divide3/1
  [TCap] -> Divide4/1
  Divide3/1 -> Saturation Dynamic1/2
  [soc] -> Chart/1(LKTSoc)
  Chart/1(SocOut) -> Divide/3
  Constant5/1 -> Divide4/2
  Divide4/1 -> Divide3/2
  soh/1 -> Divide1/3
  Constant4/1 -> Divide5/1
  Constant1/1 -> Divide5/2
  Divide5/1 -> Divide2/2
  MinMax1/1 -> Add2/1, Saturation Dynamic2/1
  Add2/1 -> [CannotUsedCap], Add/1
  Saturation Dynamic1/1 -> Chart/2(CalcSoc)
  Constant3/1 -> Saturation Dynamic1/1
  Constant/1 -> Saturation Dynamic1/3
  Divide2/1 -> Saturation Dynamic2/2
  Constant10/1 -> Saturation Dynamic2/3
  Constant42/1 -> Divide16/2
  Constant43/1 -> MinMax/1
  MinMax/1 -> Divide16/3
  Divide16/1 -> MinMax1/1
  Constant25/1 -> MinMax1/2
  Constant31/1 -> Divide16/1

== system Udan_SOC/SOC_Calculate/UdanSOCCalcn/CapAdder1/LKT/LKT_Temp20/Current_1C ==
  UCell : Inport
  Enable : EnablePort
  1-D Lookup Table : Lookup_n-D  NumberOfTableDimensions=1  BreakpointsForDimension1=uint16([4110,4118]);  Table=uint16([8500,8570]);  ExtrapMethod=Clip  UseLastTableValue=on  InternalRulePriority=Speed  OutDataTypeStr=uint16  RndMeth=Simplest
  SOC : Outport
  wires:
  UCell/1 -> 1-D Lookup Table/1
  1-D Lookup Table/1 -> SOC/1

== system Udan_SOC/SOC_Calculate/UdanSOCCalcn/CapAdder1/LKT/LKT_Temp20/Current_1C1 ==
  UCell : Inport
  Enable : EnablePort
  1-D Lookup Table2 : Lookup_n-D  NumberOfTableDimensions=1  BreakpointsForDimension1=uint16([4080,4106,4138]);  Table=uint16([8700,9000,9280]);  ExtrapMethod=Clip  UseLastTableValue=on  InternalRulePriority=Speed  OutDataTypeStr=uint16  RndMeth=Simplest
  SOC : Outport
  wires:
  UCell/1 -> 1-D Lookup Table2/1
  1-D Lookup Table2/1 -> SOC/1

== system Udan_SOC/SOC_Calculate/UdanSOCCalcn/CapAdder1/LKT/LKT_Temp40/Current_1C ==
  UCell : Inport
  Enable : EnablePort
  1-D Lookup Table1 : Lookup_n-D  NumberOfTableDimensions=1  BreakpointsForDimension1=uint16([4053,4110,4118]);  Table=uint16([8500,9000,9070]);  ExtrapMethod=Clip  UseLastTableValue=on  InternalRulePriority=Speed  OutDataTypeStr=uint16  RndMeth=Simplest
  SOC : Outport
  wires:
  UCell/1 -> 1-D Lookup Table1/1
  1-D Lookup Table1/1 -> SOC/1

== system Udan_SOC/SOC_Calculate/UdanSOCCalcn/CapAdder1/LKT/LKT_Temp40/Current_1C1 ==
  UCell : Inport
  Enable : EnablePort
  1-D Lookup Table4 : Lookup_n-D  NumberOfTableDimensions=1  BreakpointsForDimension1=uint16([4105,4138]);  Table=uint16([9200,9500]);  ExtrapMethod=Clip  UseLastTableValue=on  InternalRulePriority=Speed  OutDataTypeStr=uint16  RndMeth=Simplest
  SOC : Outport
  wires:
  UCell/1 -> 1-D Lookup Table4/1
  1-D Lookup Table4/1 -> SOC/1

== system Udan_SOC/SOC_Calculate/UdanSOCCalcn/CapAdder1/LKT/LKT_Temp45/Current_1C ==
  UCell : Inport
  Enable : EnablePort
  1-D Lookup Table5 : Lookup_n-D  NumberOfTableDimensions=1  BreakpointsForDimension1=uint16([4024,4079,4118]);  Table=uint16([8500,9000,9350]);  ExtrapMethod=Clip  UseLastTableValue=on  InternalRulePriority=Speed  OutDataTypeStr=uint16  RndMeth=Simplest
  SOC : Outport
  wires:
  UCell/1 -> 1-D Lookup Table5/1
  1-D Lookup Table5/1 -> SOC/1

== system Udan_SOC/SOC_Calculate/UdanSOCCalcn/CapAdder1/LKT/LKT_Temp45/Current_1C1 ==
  UCell : Inport
  Enable : EnablePort
  1-D Lookup Table6 : Lookup_n-D  NumberOfTableDimensions=1  BreakpointsForDimension1=uint16([4112,4118]);  Table=uint16([9400,9350]);  ExtrapMethod=Clip  UseLastTableValue=on  InternalRulePriority=Speed  OutDataTypeStr=uint16  RndMeth=Simplest
  SOC : Outport
  wires:
  UCell/1 -> 1-D Lookup Table6/1
  1-D Lookup Table6/1 -> SOC/1

== system Udan_SOC/SOC_Calculate/UdanSOCCalcn/Function-Call Subsystem4/Subsystem1/Subsystem1/Subsystem ==
  HighIndex : Inport
  LowIndex : Inport  Port=2
  Enable : EnablePort
  Add : Sum
  Bit Rotate : hdlsllib/Logic and Bit Operations/Bit Rotate  mode=Rotate Left  N=16
      settings: SourceProductName=HDL Coder  SourceProductBaseCode=HD
  Data Type Conversion : DataTypeConversion  OutDataTypeStr=uint32
  soc : Outport
  wires:
  LowIndex/1 -> Add/2
  Bit Rotate/1 -> Add/1
  Data Type Conversion/1 -> Bit Rotate/1
  HighIndex/1 -> Data Type Conversion/1
  Add/1 -> soc/1  "soc"

== system Udan_SOC/SOC_Calculate/UdanSOCCalcn/StoreCulumutiveAh/StoreChgAh/Subsystem1/Subsystem ==
  HighIndex : Inport
  LowIndex : Inport  Port=2
  Enable : EnablePort
  Add : Sum
  Bit Rotate : hdlsllib/Logic and Bit Operations/Bit Rotate  mode=Rotate Left  N=16
      settings: SourceProductName=HDL Coder  SourceProductBaseCode=HD
  Data Type Conversion : DataTypeConversion  OutDataTypeStr=uint32
  soc : Outport
  wires:
  LowIndex/1 -> Add/2
  Bit Rotate/1 -> Add/1
  Data Type Conversion/1 -> Bit Rotate/1
  HighIndex/1 -> Data Type Conversion/1
  Add/1 -> soc/1  "soc"

== system Udan_SOC/SOC_Calculate/UdanSOCCalcn/StoreCulumutiveAh/StoreDchgAh1/Subsystem1/Subsystem ==
  HighIndex : Inport
  LowIndex : Inport  Port=2
  Enable : EnablePort
  Add : Sum
  Bit Rotate : hdlsllib/Logic and Bit Operations/Bit Rotate  mode=Rotate Left  N=16
      settings: SourceProductName=HDL Coder  SourceProductBaseCode=HD
  Data Type Conversion : DataTypeConversion  OutDataTypeStr=uint32
  soc : Outport
  wires:
  LowIndex/1 -> Add/2
  Bit Rotate/1 -> Add/1
  Data Type Conversion/1 -> Bit Rotate/1
  HighIndex/1 -> Data Type Conversion/1
  Add/1 -> soc/1  "soc"
